simulink model "cp"  (R2025b)
settings: Solver=VariableStepAuto  StartTime=0.0  StopTime=5  RelTol=1e-3
settings Model: Creator=Admin  LastModifiedBy=Vishal
settings OptimizationCC: ReuseModelBlockBuffer=off
settings RTWCC: GPUComputeCapability=3.5

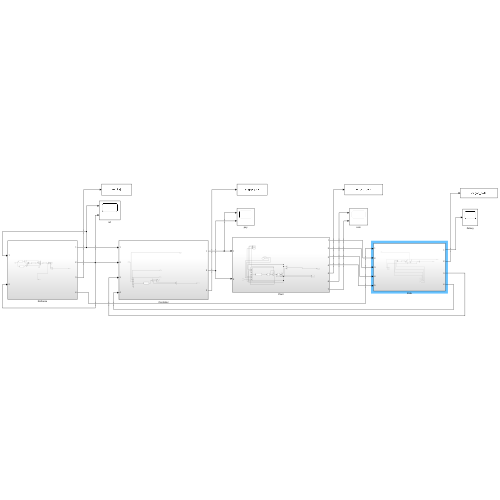
[thumbnail: Simulink's stored preview of the top-level diagram]
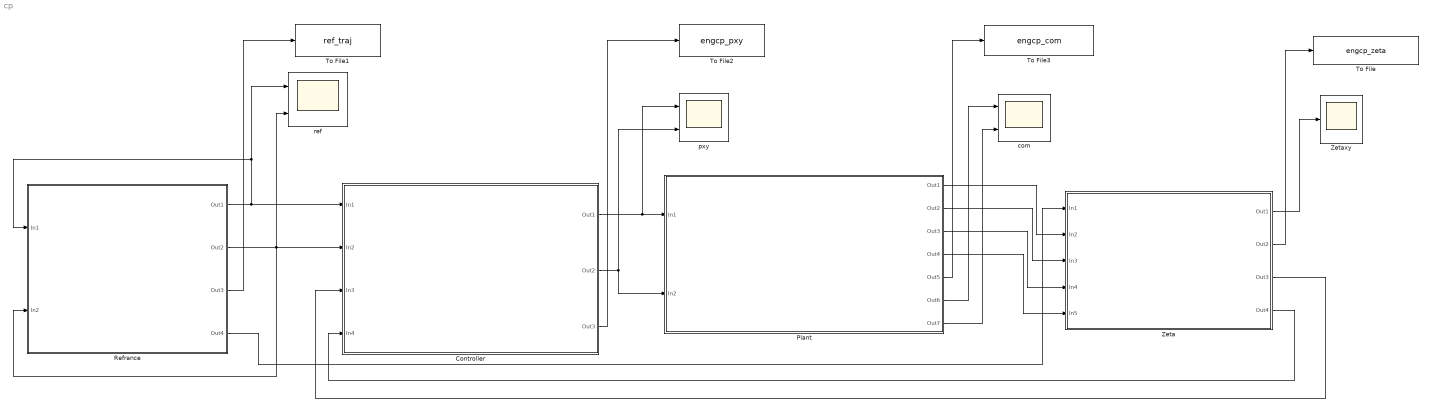
== system cp ==
  Controller : Subsystem
  Plant : Subsystem
  Refrance : Subsystem
  To File : ToFile  Filename=engcp_zeta  MatrixName=states_engd
  To File1 : ToFile  Filename=ref_traj  MatrixName=states_ref
  To File2 : ToFile  Filename=engcp_pxy  MatrixName=states_engd_px
  To File3 : ToFile  Filename=engcp_com  MatrixName=states_engd_com
  Zeta : Subsystem
  Zetaxy : Scope
      settings: ActiveDisplayYMinimum=-1  ActiveDisplayYMaximum=1
  com : Scope  NumInputPorts=2
      settings: ActiveDisplayYMinimum=-1.3763966580285247  ActiveDisplayYMaximum=1.6637793163818488
  pxy : Scope  NumInputPorts=2
      settings: ActiveDisplayYMinimum=-14.46093  ActiveDisplayYMaximum=15.60178  DataLoggingVariableName=ScopeData4
  ref : Scope  NumInputPorts=2
      settings: ActiveDisplayYMinimum=-1  ActiveDisplayYMaximum=1
  wires:
  Refrance/2(Out2) -> Refrance/2(In2), ref/2, Controller/2(In2)
  Refrance/1(Out1) -> Refrance/1(In1), ref/1, Controller/1(In1)
  Refrance/3(Out3) -> To File1/1
  Plant/5(Out5) -> To File3/1
  Plant/6(Out6) -> com/1
  Plant/7(Out7) -> com/2
  Controller/1(Out1) -> Plant/1(In1), pxy/1
  Controller/2(Out2) -> pxy/2, Plant/2(In2)
  Controller/3(Out3) -> To File2/1
  Refrance/4(Out4) -> Zeta/1(In1)
  Plant/1(Out1) -> Zeta/2(In2)
  Plant/2(Out2) -> Zeta/3(In3)
  Plant/3(Out3) -> Zeta/4(In4)
  Plant/4(Out4) -> Zeta/5(In5)
  Zeta/1(Out1) -> Zetaxy/1
  Zeta/2(Out2) -> To File/1
  Zeta/3(Out3) -> Controller/3(In3)
  Zeta/4(Out4) -> Controller/4(In4)

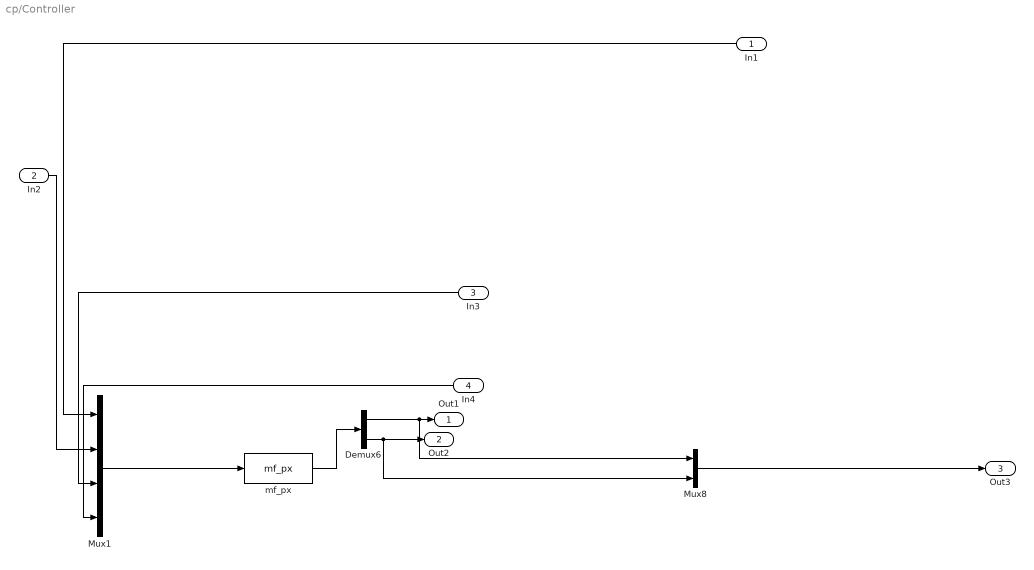
== system cp/Controller ==
  In1 : Inport
  In2 : Inport  Port=2
  In3 : Inport  Port=3
  In4 : Inport  Port=4
  Demux6 : Demux  Outputs=2
  Mux1 : Mux
  Mux8 : Mux  Inputs=2
  mf_px : MATLABFcn  MATLABFcn=mf_px  OutputDimensions=2
  Out1 : Outport
  Out2 : Outport  Port=2
  Out3 : Outport  Port=3
  wires:
  Demux6/2 -> Out2/1, Mux8/2
  In3/1 -> Mux1/3
  mf_px/1 -> Demux6/1
  Mux1/1 -> mf_px/1
  Demux6/1 -> Mux8/1, Out1/1
  Mux8/1 -> Out3/1
  In1/1 -> Mux1/1
  In2/1 -> Mux1/2
  In4/1 -> Mux1/4

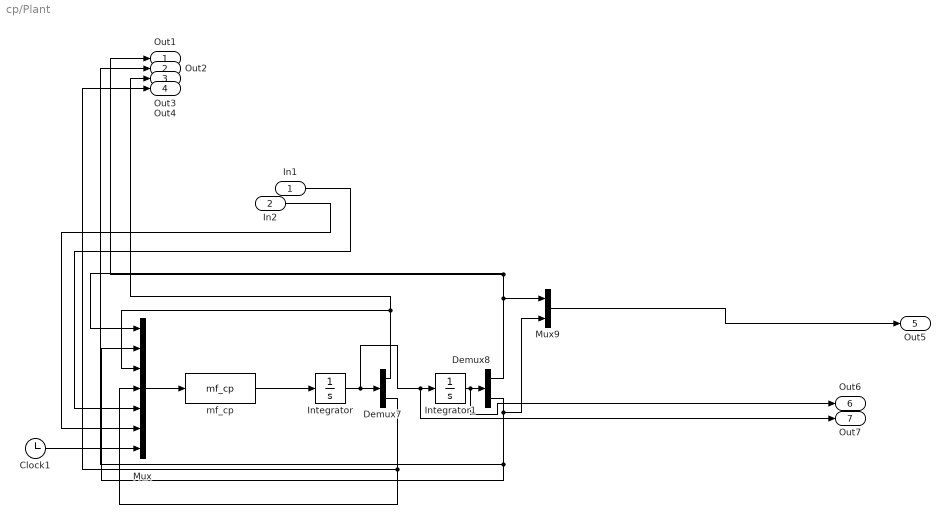
== system cp/Plant ==
  In1 : Inport
  In2 : Inport  Port=2
  Clock1 : Clock
  Demux7 : Demux  Outputs=2
  Demux8 : Demux  Outputs=2
  Integrator : Integrator  InitialCondition=0.01
  Integrator1 : Integrator
  Mux : Mux  Inputs=7
  Mux9 : Mux  Inputs=2
  mf_cp : MATLABFcn  MATLABFcn=mf_cp  OutputDimensions=2
  Out1 : Outport
  Out2 : Outport  Port=2
  Out3 : Outport  Port=3
  Out4 : Outport  Port=4
  Out5 : Outport  Port=5
  Out6 : Outport  Port=6
  Out7 : Outport  Port=7
  wires:
  Mux9/1 -> Out5/1
  Demux8/2 -> Mux9/2, Out2/1, Mux/2
  Demux8/1 -> Out1/1, Mux/1, Mux9/1
  Clock1/1 -> Mux/7
  Integrator1/1 -> Out6/1, Demux8/1
  Demux7/2 -> Out4/1, Mux/4
  Integrator/1 -> Out7/1, Integrator1/1, Demux7/1
  In1/1 -> Mux/5
  mf_cp/1 -> Integrator/1
  Demux7/1 -> Out3/1, Mux/3
  Mux/1 -> mf_cp/1
  In2/1 -> Mux/6

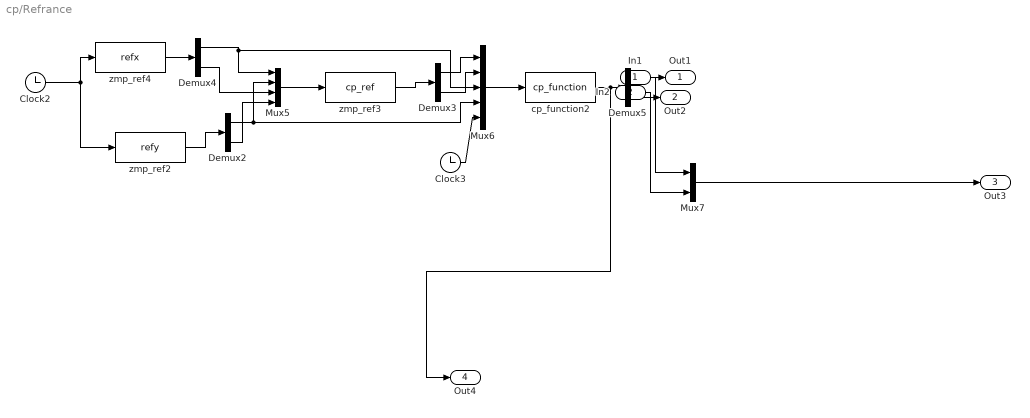
== system cp/Refrance ==
  In1 : Inport
  In2 : Inport  Port=2
  Clock2 : Clock
  Clock3 : Clock
  Demux{2..5} (4 alike) : Demux  Outputs=2
  Mux5 : Mux
  Mux6 : Mux  Inputs=5
  Mux7 : Mux  Inputs=2
  cp_function2 : MATLABFcn  MATLABFcn=cp_function  OutputDimensions=2
  zmp_ref2 : MATLABFcn  MATLABFcn=refy
  zmp_ref3 : MATLABFcn  MATLABFcn=cp_ref  OutputDimensions=2
  zmp_ref4 : MATLABFcn  MATLABFcn=refx
  Out1 : Outport
  Out2 : Outport  Port=2
  Out3 : Outport  Port=3
  Out4 : Outport  Port=4
  wires:
  zmp_ref4/1 -> Demux4/1
  Demux2/2 -> Mux5/4
  Mux5/1 -> zmp_ref3/1
  Demux2/1 -> Mux6/4, Mux5/2
  zmp_ref2/1 -> Demux2/1
  Demux3/1 -> Mux6/1
  Mux6/1 -> cp_function2/1
  Clock3/1 -> Mux6/5
  In2/1 -> Mux7/2
  Demux3/2 -> Mux6/2
  In1/1 -> Mux7/1
  Mux7/1 -> Out3/1
  zmp_ref3/1 -> Demux3/1
  cp_function2/1 -> Out4/1, Demux5/1
  Demux4/2 -> Mux5/3
  Clock2/1 -> zmp_ref4/1, zmp_ref2/1
  Demux4/1 -> Mux6/3, Mux5/1
  Demux5/1 -> Out1/1
  Demux5/2 -> Out2/1

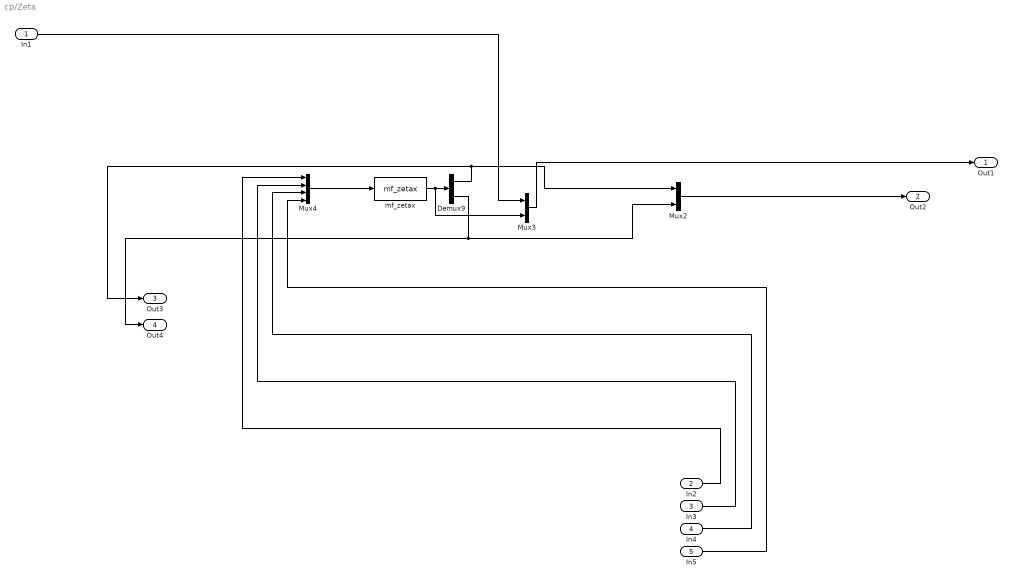
== system cp/Zeta ==
  In1 : Inport
  In2 : Inport  Port=2
  In3 : Inport  Port=3
  In4 : Inport  Port=4
  In5 : Inport  Port=5
  Demux9 : Demux  Outputs=2
  Mux2 : Mux  Inputs=2
  Mux3 : Mux  Inputs=2
  Mux4 : Mux
  mf_zetax : MATLABFcn  MATLABFcn=mf_zetax  OutputDimensions=2
  Out1 : Outport
  Out2 : Outport  Port=2
  Out3 : Outport  Port=3
  Out4 : Outport  Port=4
  wires:
  Demux9/1 -> Out3/1, Mux2/1
  Demux9/2 -> Out4/1, Mux2/2
  Mux2/1 -> Out2/1
  Mux4/1 -> mf_zetax/1
  mf_zetax/1 -> Mux3/2, Demux9/1
  In4/1 -> Mux4/3
  In1/1 -> Mux3/1
  Mux3/1 -> Out1/1
  In2/1 -> Mux4/1
  In5/1 -> Mux4/4
  In3/1 -> Mux4/2
